simulink model "torqueWalkingR2017a"  (Simulink 9.0)
settings: Solver=FixedStepDiscrete  StartTime=0.0  StopTime=Config.t_end  FixedStep=Config.t_step  RelTol=1e-3  EnableMultiTasking=on
InitFcn:
  | cd(fileparts(which(bdroot)));
  | initTorqueWalking;
StopFcn:
  | cd(fileparts(which(bdroot)));
  | disp_early_termination
undefined symbols (not defined in the file or in its folder): biasVectorConstraint_feet, Config, CONFIG, ConstraintMatrix_feet, DiscIntNeverNeededParam, Gains, ROBOT_DOF, Sat
libraries: WBToolboxLibrary x113, commchan3 x2, simulink x2
(part 4 of 4)

== system torqueWalkingR2017a/Robot State and References/Smooth References /Smooth Reference Orientations/Compute Smoothed Ref Orientations ==
  w_R_LFoot_des : Inport
  w_R_RFoot_des : Inport  Port=2
  w_R_rot_task_des : Inport  Port=3
  w_R_LHand_des : Inport  Port=4
  w_R_RHand_des : Inport  Port=5
  omega_LFoot : Inport  Port=6
  omega_RFoot : Inport  Port=7
  omega_rot_task : Inport  Port=8
  omega_LHand : Inport  Port=9
  omega_RHand : Inport  Port=10
  Compute Rotation Matrix Derivative : MATLAB Function  TreatAsAtomicUnit=on
  Discrete-Time Integrator{1..5} (5 alike) : DiscreteIntegrator  InitialConditionSource=external  InitialCondition=zeros(3,1)  InitialConditionSetting=State (most efficient)  SampleTime=Config.t_step  ICPrevOutput=DiscIntNeverNeededParam  ICPrevScaledInput=DiscIntNeverNeededParam
  holder {,1..4} (5 alike) : WBToolboxLibrary/Utilities/holder 
      settings: SourceProductName=Whole Body Toolbox
  w_R_LFoot : Outport
  w_R_RFoot : Outport  Port=2
  w_R_rot_task : Outport  Port=3
  w_R_LHand : Outport  Port=4
  w_R_RHand : Outport  Port=5
  wires:
  "holder "/1 -> Discrete-Time Integrator2/2
  holder 2/1 -> Discrete-Time Integrator5/2
  holder 1/1 -> Discrete-Time Integrator1/2
  Compute Rotation Matrix Derivative/1(RDot_LFoot) -> Discrete-Time Integrator2/1
  Compute Rotation Matrix Derivative/2(RDot_RFoot) -> Discrete-Time Integrator5/1
  Compute Rotation Matrix Derivative/3(RDot_rot_task) -> Discrete-Time Integrator1/1
  w_R_LFoot_des/1 -> "holder "/1
  w_R_RFoot_des/1 -> holder 2/1
  w_R_rot_task_des/1 -> holder 1/1
  Discrete-Time Integrator2/1 -> w_R_LFoot/1, Compute Rotation Matrix Derivative/6(w_R_LFoot)
  Discrete-Time Integrator1/1 -> w_R_rot_task/1, Compute Rotation Matrix Derivative/8(w_R_rot_task)
  omega_LFoot/1 -> Compute Rotation Matrix Derivative/1(omega_LFoot)
  omega_RFoot/1 -> Compute Rotation Matrix Derivative/2(omega_RFoot)
  omega_rot_task/1 -> Compute Rotation Matrix Derivative/3(omega_rot_task)
  Discrete-Time Integrator5/1 -> w_R_RFoot/1, Compute Rotation Matrix Derivative/7(w_R_RFoot)
  omega_LHand/1 -> Compute Rotation Matrix Derivative/4(omega_LHand)
  omega_RHand/1 -> Compute Rotation Matrix Derivative/5(omega_RHand)
  Discrete-Time Integrator4/1 -> w_R_RHand/1, Compute Rotation Matrix Derivative/10(w_R_RHand)
  Discrete-Time Integrator3/1 -> w_R_LHand/1, Compute Rotation Matrix Derivative/9(w_R_LHand)
  w_R_RHand_des/1 -> holder 4/1
  w_R_LHand_des/1 -> holder 3/1
  Compute Rotation Matrix Derivative/5(RDot_RHand) -> Discrete-Time Integrator4/1
  Compute Rotation Matrix Derivative/4(RDot_LHand) -> Discrete-Time Integrator3/1
  holder 4/1 -> Discrete-Time Integrator4/2
  holder 3/1 -> Discrete-Time Integrator3/2

== system torqueWalkingR2017a/Robot State and References/State Machines/Compute Feet to Base Link Transforms/LFoot to base link transform  ==
  s : Inport
  inertial : Inport  Port=2
  w_H_link : Inport  Port=3
  w_H_base_fixed : Inport  Port=4
  Fixed base to imu transform : WBToolboxLibrary/wholeBodyModel/Kinematics/Forward Kinematics  frameName=Frames.IMU
      settings: SourceProductName=Whole Body Toolbox
  Fixed base to root link transform : WBToolboxLibrary/wholeBodyModel/Kinematics/Forward Kinematics  frameName=Frames.BASE_LINK
      settings: SourceProductName=Whole Body Toolbox
  Inv\* : Product  Inputs=/*  Multiplication=Matrix(*)
  "Inv\\*  " : Product  Inputs=/*  Multiplication=Matrix(*)
  Neck Position : WBToolboxLibrary/Utilities/Yarp Read  portName=Ports.NECK_POS  signalSize=6  timeout=0.5  blocking=off  timestamp=off  autoconnect=on  errorOnConnection=off
      settings: SourceProductName=Whole Body Toolbox
  Switch6 : Switch  Criteria=u2 > Threshold
  USE_IMU4EST_BASE : Constant  Value=Config.USE_IMU4EST_BASE
  fromImuToHomogeousTransformFCN : MATLAB Function  TreatAsAtomicUnit=on
  holder 1 : WBToolboxLibrary/Utilities/holder 
      settings: SourceProductName=Whole Body Toolbox
  holder 2 : WBToolboxLibrary/Utilities/holder 
      settings: SourceProductName=Whole Body Toolbox
  neck transform : Subsystem
  link_H_b : Outport
  wires:
  Switch6/1 -> link_H_b/1
  "Inv\\*  "/1 -> Switch6/3, fromImuToHomogeousTransformFCN/3(link_H_base)  "link_H_root"
  USE_IMU4EST_BASE/1 -> Switch6/2
  Inv\*/1 -> fromImuToHomogeousTransformFCN/1(imu_H_link), holder 1/1  "imu_H_link"
  holder 2/1 -> fromImuToHomogeousTransformFCN/4(inertial_0)
  Fixed base to imu transform/1 -> Inv\*/1
  holder 1/1 -> fromImuToHomogeousTransformFCN/2(imu_H_link_0)
  s/1 -> Fixed base to imu transform/2, Fixed base to root link transform/2
  fromImuToHomogeousTransformFCN/1(w_H_b) -> Switch6/1
  Fixed base to root link transform/1 -> "Inv\\*  "/2
  inertial/1 -> holder 2/1, fromImuToHomogeousTransformFCN/5(inertial)
  Neck Position/1 -> neck transform/1(neck port)
  neck transform/1(neck position) -> fromImuToHomogeousTransformFCN/6(neck_pos)
  w_H_link/1 -> "Inv\\*  "/1, Inv\*/2
  w_H_base_fixed/1 -> Fixed base to root link transform/1, Fixed base to imu transform/1

== system torqueWalkingR2017a/Robot State and References/State Machines/Compute Feet to Base Link Transforms/RFoot to base link transform ==
  s : Inport
  inertial : Inport  Port=2
  w_H_link : Inport  Port=3
  w_H_base_fixed : Inport  Port=4
  Fixed base to imu transform : WBToolboxLibrary/wholeBodyModel/Kinematics/Forward Kinematics  frameName=Frames.IMU
      settings: SourceProductName=Whole Body Toolbox
  Fixed base to root link transform : WBToolboxLibrary/wholeBodyModel/Kinematics/Forward Kinematics  frameName=Frames.BASE_LINK
      settings: SourceProductName=Whole Body Toolbox
  Inv\* : Product  Inputs=/*  Multiplication=Matrix(*)
  "Inv\\*  " : Product  Inputs=/*  Multiplication=Matrix(*)
  Neck Position : WBToolboxLibrary/Utilities/Yarp Read  portName=Ports.NECK_POS  signalSize=6  timeout=0.5  blocking=off  timestamp=off  autoconnect=on  errorOnConnection=off
      settings: SourceProductName=Whole Body Toolbox
  Switch6 : Switch  Criteria=u2 > Threshold
  USE_IMU4EST_BASE : Constant  Value=Config.USE_IMU4EST_BASE
  fromImuToHomogeousTransformFCN : MATLAB Function  TreatAsAtomicUnit=on
  holder 1 : WBToolboxLibrary/Utilities/holder 
      settings: SourceProductName=Whole Body Toolbox
  holder 2 : WBToolboxLibrary/Utilities/holder 
      settings: SourceProductName=Whole Body Toolbox
  neck transform : Subsystem
  link_H_b : Outport
  wires:
  Switch6/1 -> link_H_b/1
  "Inv\\*  "/1 -> Switch6/3, fromImuToHomogeousTransformFCN/3(link_H_base)  "link_H_root"
  USE_IMU4EST_BASE/1 -> Switch6/2
  Inv\*/1 -> fromImuToHomogeousTransformFCN/1(imu_H_link), holder 1/1  "imu_H_link"
  holder 2/1 -> fromImuToHomogeousTransformFCN/4(inertial_0)
  Fixed base to imu transform/1 -> Inv\*/1
  holder 1/1 -> fromImuToHomogeousTransformFCN/2(imu_H_link_0)
  s/1 -> Fixed base to imu transform/2, Fixed base to root link transform/2
  fromImuToHomogeousTransformFCN/1(w_H_b) -> Switch6/1
  Fixed base to root link transform/1 -> "Inv\\*  "/2
  inertial/1 -> holder 2/1, fromImuToHomogeousTransformFCN/5(inertial)
  Neck Position/1 -> neck transform/1(neck port)
  neck transform/1(neck position) -> fromImuToHomogeousTransformFCN/6(neck_pos)
  w_H_link/1 -> "Inv\\*  "/1, Inv\*/2
  w_H_base_fixed/1 -> Fixed base to root link transform/1, Fixed base to imu transform/1

== system torqueWalkingR2017a/Robot State and References/State Machines/Compute State Velocity/Feet Jacobians ==
  s : Inport
  w_H_b : Inport  Port=2
  Jacobian LFoot : WBToolboxLibrary/wholeBodyModel/Jacobians/Jacobian  frameName=Frames.LEFT_FOOT
      settings: SourceProductName=Whole Body Toolbox
  Jacobian RFoot : WBToolboxLibrary/wholeBodyModel/Jacobians/Jacobian  frameName=Frames.RIGHT_FOOT
      settings: SourceProductName=Whole Body Toolbox
  J_LFoot : Outport
  J_RFoot : Outport  Port=2
  wires:
  Jacobian LFoot/1 -> J_LFoot/1
  Jacobian RFoot/1 -> J_RFoot/1
  w_H_b/1 -> Jacobian RFoot/1, Jacobian LFoot/1
  s/1 -> Jacobian LFoot/2, Jacobian RFoot/2

== system torqueWalkingR2017a/Robot State and References/State Machines/Select the Current State and References/task position and orientation ==
  s : Inport
  w_H_b : Inport  Port=2
  CoM : WBToolboxLibrary/wholeBodyModel/Kinematics/Forward Kinematics  frameName=Frames.COM
      settings: SourceProductName=Whole Body Toolbox
  LArm : WBToolboxLibrary/wholeBodyModel/Kinematics/Forward Kinematics  frameName=Frames.LEFT_HAND
      settings: SourceProductName=Whole Body Toolbox
  LFoot : WBToolboxLibrary/wholeBodyModel/Kinematics/Forward Kinematics  frameName=Frames.LEFT_FOOT
      settings: SourceProductName=Whole Body Toolbox
  RArm : WBToolboxLibrary/wholeBodyModel/Kinematics/Forward Kinematics  frameName=Frames.RIGHT_HAND
      settings: SourceProductName=Whole Body Toolbox
  RFoot : WBToolboxLibrary/wholeBodyModel/Kinematics/Forward Kinematics  frameName=Frames.RIGHT_FOOT
      settings: SourceProductName=Whole Body Toolbox
  rotational task : WBToolboxLibrary/wholeBodyModel/Kinematics/Forward Kinematics  frameName=Frames.ROT_TASK_LINK
      settings: SourceProductName=Whole Body Toolbox
  w_H_l_sole : Outport
  w_H_r_sole : Outport  Port=2
  w_H_CoM : Outport  Port=3
  w_H_rot_task : Outport  Port=4
  w_H_l_hand : Outport  Port=5
  w_H_r_hand : Outport  Port=6
  wires:
  s/1 -> RArm/2, LArm/2, rotational task/2, CoM/2, RFoot/2, LFoot/2
  w_H_b/1 -> RArm/1, LArm/1, rotational task/1, CoM/1, LFoot/1, RFoot/1
  CoM/1 -> w_H_CoM/1
  LFoot/1 -> w_H_l_sole/1
  RFoot/1 -> w_H_r_sole/1
  rotational task/1 -> w_H_rot_task/1
  LArm/1 -> w_H_l_hand/1
  RArm/1 -> w_H_r_hand/1

== system torqueWalkingR2017a/Robot State and References/State Machines/Compute Feet to Base Link Transforms/LFoot to base link transform /neck transform ==
  neck port : Inport
  Constant : Constant  Value=zeros(3,1)
  Gain : Gain  Gain=pi/180
  Selector1 : Selector  InputPortWidth=6  IndexOptions=Index vector (dialog)  Indices=[1:3]  OutputSizes=1
  Switch : Switch  Criteria=u2 > Threshold
  USE_IMU4EST_BASE1 : Constant  Value=Config.CORRECT_IMU_WITH_NECK_POS
  neck position : Outport
  wires:
  neck port/1 -> Gain/1
  USE_IMU4EST_BASE1/1 -> Switch/2
  Switch/1 -> neck position/1
  Gain/1 -> Selector1/1
  Constant/1 -> Switch/3
  Selector1/1 -> Switch/1  "neck pos"

== system torqueWalkingR2017a/Robot State and References/State Machines/Compute Feet to Base Link Transforms/RFoot to base link transform/neck transform ==
  neck port : Inport
  Constant : Constant  Value=zeros(3,1)
  Gain : Gain  Gain=pi/180
  Selector1 : Selector  InputPortWidth=6  IndexOptions=Index vector (dialog)  Indices=[1:3]  OutputSizes=1
  Switch : Switch  Criteria=u2 > Threshold
  USE_IMU4EST_BASE1 : Constant  Value=Config.CORRECT_IMU_WITH_NECK_POS
  neck position : Outport
  wires:
  neck port/1 -> Gain/1
  USE_IMU4EST_BASE1/1 -> Switch/2
  Switch/1 -> neck position/1
  Gain/1 -> Selector1/1
  Constant/1 -> Switch/3
  Selector1/1 -> Switch/1  "neck pos"

== matlab function Dynamics and Kinematics/Initial Conditions/compute state velocity/Compute Base Velocity ==
  data: J_LeftFoot input double; J_RightFoot input double; feetInContact input double; nu_b output double; sDot input double; Sat parameter double
function nu_b = computeBaseVelocityFCN(J_LeftFoot, J_RightFoot, feetInContact, sDot, Sat)

    nu_b = computeBaseVelocity(J_LeftFoot, J_RightFoot, feetInContact, sDot, Sat);
end

== matlab function Balancing Controller (Reactive QP control)/Balancing Controller Function ==
  data: feetInContact input double; M input double; Hessian output double; h input double; J input double; impedances input double; dampings input double; s input double; sDot input double; s_sDot_sDDot_des input double; acc_task_star input double; JDot_nu input double; ConstraintsMatrix_feet input double; biasVectorConstraint_feet input double; w_H_l_sole input double; w_H_r_sole input double; gradient output double; ConstraintMatrix_equality output double; biasVectorConstraint_equality output double; ConstraintMatrix_inequality output double; biasVectorConstraint_inequality output double; Sat parameter double; Config parameter double; ROBOT_DOF parameter double
function [Hessian,gradient,ConstraintMatrix_equality,biasVectorConstraint_equality, ...
          ConstraintMatrix_inequality,biasVectorConstraint_inequality] = ...
          balancingControllerFCN(feetInContact, M, h, J, impedances, ...
                                 dampings, s, sDot, s_sDot_sDDot_des, acc_task_star, ...
                                 JDot_nu, ConstraintsMatrix_feet, biasVectorConstraint_feet, ...
                                 w_H_l_sole, w_H_r_sole, Sat, Config, ROBOT_DOF)
                          

    [Hessian,gradient,ConstraintMatrix_equality,biasVectorConstraint_equality, ...
     ConstraintMatrix_inequality,biasVectorConstraint_inequality] = ...
         balancingController(feetInContact, M, h, J, impedances, ...
                                dampings, s, sDot, s_sDot_sDDot_des, acc_task_star, ...
                                JDot_nu, ConstraintsMatrix_feet, biasVectorConstraint_feet, ...
                                w_H_l_sole, w_H_r_sole, Sat, Config, ROBOT_DOF);                         
end

== matlab function Dynamics and Kinematics/Inverse Kinematics/Compute tasks accelerations ==
  data: pose_vel_acc_LFoot_des input double; pose_vel_acc_RFoot_des input double; pos_vel_acc_CoM_des input double; acc_task_star output double; orient_vel_acc_rot_task_des input double; pose_vel_acc_LHand_des input double; pose_vel_acc_RHand_des input double; pose_vel_LFoot input double; pose_vel_RFoot input double; pos_vel_CoM input double; orient_vel_rot_task input double; pose_vel_LHand input double; pose_vel_RHand input double; Kp_Kd_LFoot input double; Kp_Kd_RFoot input double; Kp_Kd_CoM input double; Kp_Kd_rot_task input double; Kp_Kd_LHand input double; Kp_Kd_RHand input double; feetInContact input double; Sat parameter double
function acc_task_star = setTasksAccelerationsFCN(pose_vel_acc_LFoot_des, pose_vel_acc_RFoot_des, pos_vel_acc_CoM_des, orient_vel_acc_rot_task_des, pose_vel_acc_LHand_des,pose_vel_acc_RHand_des, ...
                                                  pose_vel_LFoot, pose_vel_RFoot, pos_vel_CoM, orient_vel_rot_task, pose_vel_LHand, pose_vel_RHand, ...
                                                  Kp_Kd_LFoot, Kp_Kd_RFoot, Kp_Kd_CoM, Kp_Kd_rot_task, Kp_Kd_LHand, Kp_Kd_RHand,...
                                                  feetInContact, Sat) 

    acc_task_star = setTasksAccelerations(pos_vel_acc_CoM_des, pose_vel_acc_LFoot_des, pose_vel_acc_RFoot_des, orient_vel_acc_rot_task_des, pose_vel_acc_LHand_des,pose_vel_acc_RHand_des, ...
                                          pos_vel_CoM, pose_vel_LFoot, pose_vel_RFoot, orient_vel_rot_task, pose_vel_LHand, pose_vel_RHand, ...
                                          Kp_Kd_CoM, Kp_Kd_LFoot, Kp_Kd_RFoot, Kp_Kd_rot_task, Kp_Kd_LHand, Kp_Kd_RHand,...
                                          feetInContact, Sat) ; 
                                      
                                      
end

== matlab function Dynamics and Kinematics/Inverse Kinematics/ComputeTasksPoseAndVelocity/Compose Task Pose and Velocity ==
  data: vel_LFoot input double; vel_RFoot input double; pose_vel_LFoot output double; pose_vel_RFoot output double; vel_CoM input double; vel_rot_task input double; vel_LHand input double; vel_RHand input double; w_H_l_sole input double; w_H_r_sole input double; pos_vel_CoM output double; orient_vel_rot_task output double; w_H_CoM input double; w_H_rot_task input double; w_H_l_hand input double; w_H_r_hand input double; pose_vel_LHand output double; pose_vel_RHand output double
function [pose_vel_LFoot, pose_vel_RFoot, pos_vel_CoM, orient_vel_rot_task, pose_vel_LHand, pose_vel_RHand] = ...
             composeTaskPoseAndVelocityFCN(vel_LFoot, vel_RFoot, vel_CoM, vel_rot_task, vel_LHand, vel_RHand, ...
                                           w_H_l_sole, w_H_r_sole, w_H_CoM, w_H_rot_task, w_H_l_hand, w_H_r_hand)
                                                                                                                              
    [pos_vel_CoM, pose_vel_LFoot, pose_vel_RFoot, orient_vel_rot_task, pose_vel_LHand, pose_vel_RHand] = ...
        composeTaskPoseAndVelocity(vel_CoM, vel_LFoot, vel_RFoot, vel_rot_task, vel_LHand, vel_RHand, ...
                                   w_H_CoM, w_H_l_sole, w_H_r_sole, w_H_rot_task, w_H_l_hand, w_H_r_hand);
end

== matlab function Dynamics and Kinematics/Inverse Kinematics/QP-Based Inverse Kinematics/Compute QP Hessian, gradient and constraints  ==
  data: s input double; nu input double; s_sDot_sDDot_ref input double; Hessian output double; impedances input double; dampings input double; J input double; JDot_nu input double; acc_task_star input double; feetInContact input double; gradient output double; ConstraintMatrix output double; biasVectorConstraint output double; Config parameter double; Sat parameter double
function [Hessian, gradient, ConstraintMatrix, biasVectorConstraint] = ...
             computeQPHessianAndConstraintsFCN(s, nu, s_sDot_sDDot_ref, impedances, dampings, J, JDot_nu, acc_task_star, feetInContact, Config, Sat)
         
    [Hessian, gradient, ConstraintMatrix, biasVectorConstraint] = ...
        computeQPHessianAndConstraints(s, nu, s_sDot_sDDot_ref, impedances, dampings, J, JDot_nu, acc_task_star, feetInContact, Sat, Config);
end

== matlab function Dynamics and Kinematics/Task Accelerations/Compute tasks accelerations ==
  data: pos_vel_acc_CoM_des input double; acc_task_star output double; pose_vel_acc_LFoot_des input double; pose_vel_acc_RFoot_des input double; orient_vel_acc_rot_task_des input double; pose_vel_acc_LHand_des input double; pose_vel_acc_RHand_des input double; pos_vel_CoM input double; pose_vel_LFoot input double; pose_vel_RFoot input double; orient_vel_rot_task input double; pose_vel_LHand input double; pose_vel_RHand input double; Kp_Kd_CoM input double; Kp_Kd_LFoot input double; Kp_Kd_RFoot input double; Kp_Kd_rot_task input double; Kp_Kd_LHand input double; Kp_Kd_RHand input double; feetInContact input double; Sat parameter double
function acc_task_star = setTasksAccelerationsFCN(pos_vel_acc_CoM_des, pose_vel_acc_LFoot_des, pose_vel_acc_RFoot_des, orient_vel_acc_rot_task_des, pose_vel_acc_LHand_des,pose_vel_acc_RHand_des, ...
                                                  pos_vel_CoM, pose_vel_LFoot, pose_vel_RFoot, orient_vel_rot_task, pose_vel_LHand, pose_vel_RHand, ...
                                                  Kp_Kd_CoM, Kp_Kd_LFoot, Kp_Kd_RFoot, Kp_Kd_rot_task, Kp_Kd_LHand, Kp_Kd_RHand,...
                                                  feetInContact, Sat) 

    acc_task_star = setTasksAccelerations(pos_vel_acc_CoM_des, pose_vel_acc_LFoot_des, pose_vel_acc_RFoot_des, orient_vel_acc_rot_task_des, pose_vel_acc_LHand_des,pose_vel_acc_RHand_des, ...
                                          pos_vel_CoM, pose_vel_LFoot, pose_vel_RFoot, orient_vel_rot_task, pose_vel_LHand, pose_vel_RHand, ...
                                          Kp_Kd_CoM, Kp_Kd_LFoot, Kp_Kd_RFoot, Kp_Kd_rot_task, Kp_Kd_LHand, Kp_Kd_RHand,...
                                          feetInContact, Sat);

end

== matlab function Dynamics and Kinematics/Task Accelerations/ComputeTasksPoseAndVelocity/Compose Task Pose and Velocity ==
  data: vel_CoM input double; vel_LFoot input double; vel_RFoot input double; vel_rot_task input double; vel_LHand input double; vel_RHand input double; pos_vel_CoM output double; pose_vel_LFoot output double; pose_vel_RFoot output double; orient_vel_rot_task output double; w_H_CoM input double; w_H_l_sole input double; w_H_r_sole input double; w_H_rot_task input double; w_H_l_hand input double; w_H_r_hand input double; pose_vel_LHand output double; pose_vel_RHand output double
function [pos_vel_CoM, pose_vel_LFoot, pose_vel_RFoot, orient_vel_rot_task, pose_vel_LHand, pose_vel_RHand] = ...
             composeTaskPoseAndVelocityFCN(vel_CoM, vel_LFoot, vel_RFoot, vel_rot_task, vel_LHand, vel_RHand, ...
                                           w_H_CoM, w_H_l_sole, w_H_r_sole, w_H_rot_task, w_H_l_hand, w_H_r_hand)
                                                                                                                              
    [pos_vel_CoM, pose_vel_LFoot, pose_vel_RFoot, orient_vel_rot_task, pose_vel_LHand, pose_vel_RHand] = ...
        composeTaskPoseAndVelocity(vel_CoM, vel_LFoot, vel_RFoot, vel_rot_task, vel_LHand, vel_RHand, ...
                                   w_H_CoM, w_H_l_sole, w_H_r_sole, w_H_rot_task, w_H_l_hand, w_H_r_hand);
end

== matlab function Robot State and References/Gain Scheduling/Gain Scheduling Function ==
  data: state input double; Kp_CoM output double; Kd_CoM output double; Kp_LFoot output double; Kd_LFoot output double; Kp_RFoot output double; Kd_RFoot output double; Kp_rot_task output double; Kd_rot_task output double; Kp_LHand output double; Kd_LHand output double; Kp_RHand output double; Kd_RHand output double; impedances output double; dampings output double; Gains parameter double; smoothingTimeGains output double; Config parameter double
function [Kp_CoM, Kd_CoM, Kp_LFoot, Kd_LFoot, Kp_RFoot, Kd_RFoot, Kp_rot_task, Kd_rot_task, Kp_LHand, Kd_LHand, Kp_RHand, Kd_RHand, impedances, dampings, smoothingTimeGains] = ...
             gainSchedulingFCN(state,Gains,Config)

    [Kp_CoM, Kd_CoM, Kp_LFoot, Kd_LFoot, Kp_RFoot, Kd_RFoot, Kp_rot_task, Kd_rot_task, Kp_LHand, Kd_LHand, Kp_RHand, Kd_RHand, impedances, dampings, smoothingTimeGains] = ...
        gainScheduling(state,Gains,Config);
end

== matlab function Robot State and References/Smooth References /Smooth Reference Orientations/Compute Ref Ang Velocities and Accelerations/Compute Reference Angular Accelerations ==
  data: w_R_LFoot_des input double; w_R_RFoot_des input double; w_R_rot_task_des input double; w_R_LHand_des input double; w_R_RHand_des input double; w_R_LFoot input double; w_R_RFoot input double; omegaDot_LFoot output double; omegaDot_RFoot output double; omegaDot_rot_task output double; w_R_rot_task input double; w_R_LHand input double; w_R_RHand input double; state input double; omega_LFoot input double; omega_RFoot input double; omega_rot_task input double; omega_LHand input double; omega_RHand input double; Config parameter double; omegaDot_LHand output double; omegaDot_RHand output double
function [omegaDot_LFoot, omegaDot_RFoot, omegaDot_rot_task, omegaDot_LHand, omegaDot_RHand] = computeRefAngAccelerationFCN(w_R_LFoot_des, w_R_RFoot_des, w_R_rot_task_des, w_R_LHand_des, w_R_RHand_des, ...
                                                                                            w_R_LFoot, w_R_RFoot, w_R_rot_task, w_R_LHand, w_R_RHand, ...
                                                                                            state, omega_LFoot, omega_RFoot, omega_rot_task, omega_LHand, omega_RHand, Config)
         
    % Compute reference angular accelerations given a desired rotation matrix
    omegaDot_LFoot     = rotationalPID(w_R_LFoot, omega_LFoot, w_R_LFoot_des, zeros(3,1), zeros(3,1), ...
                                       Config.LFoot_Kp_smoothing(state), Config.LFoot_Kd_smoothing(state));
                                   
    omegaDot_RFoot     = rotationalPID(w_R_RFoot, omega_RFoot, w_R_RFoot_des, zeros(3,1), zeros(3,1), ...
                                       Config.RFoot_Kp_smoothing(state), Config.RFoot_Kd_smoothing(state));
                                   
    omegaDot_rot_task  = rotationalPID(w_R_rot_task, omega_rot_task, w_R_rot_task_des, zeros(3,1), zeros(3,1), ...
                                       Config.rot_task_Kp_smoothing(state), Config.rot_task_Kd_smoothing(state));

    omegaDot_LHand     = rotationalPID(w_R_LHand, omega_LHand, w_R_LHand_des, zeros(3,1), zeros(3,1), ...
                                       Config.LHand_Kp_smoothing(state), Config.LHand_Kd_smoothing(state));
                                   
    omegaDot_RHand     = rotationalPID(w_R_RHand, omega_RHand, w_R_RHand_des, zeros(3,1), zeros(3,1), ...
                                       Config.RHand_Kp_smoothing(state), Config.RHand_Kd_smoothing(state));

end

== matlab function Robot State and References/State Machines/Select the Current State and References/STATE MACHINES ==
  data: w_H_b output double; feetInContact output double; s_0 input double; w_H_LFoot input double; w_H_LFoot_0 input double; w_H_RFoot input double; w_H_RFoot_0 input double; w_H_CoM input double; w_H_CoM_0 input double; w_H_rot_task_0 input double; w_H_LHand_0 input double; w_H_RHand_0 input double; LFoot_H_b input double; RFoot_H_b input double; LFoot_wrench input double; RFoot_wrench input double; t input double; state output double; references_LFoot output double; references_RFoot output double; references_CoM output double; references_rot_task output double; references_LHand output double; references_RHand output double; references_s output double; Config parameter double; Sat parameter double
function [w_H_b, feetInContact, state, references_LFoot, references_RFoot, references_CoM, ...
          references_rot_task, references_LHand, references_RHand, references_s] = stateMachinesFCN ...
             (s_0, w_H_LFoot, w_H_LFoot_0, w_H_RFoot, w_H_RFoot_0, w_H_CoM, w_H_CoM_0, w_H_rot_task_0, ...
              w_H_LHand_0, w_H_RHand_0, LFoot_H_b, RFoot_H_b, LFoot_wrench, RFoot_wrench, t, Config, Sat)

    [w_H_b, feetInContact, state, references_LFoot, references_RFoot, references_CoM, ...
     references_rot_task, references_LHand, references_RHand, references_s] = stateMachineWalkingInPlace ...
        (s_0, w_H_LFoot, w_H_LFoot_0, w_H_RFoot, w_H_RFoot_0, w_H_CoM, w_H_CoM_0, w_H_rot_task_0, ...
         w_H_LHand_0, w_H_RHand_0, LFoot_H_b, RFoot_H_b, LFoot_wrench, RFoot_wrench, t, Config, Sat);

end

== matlab function Robot State and References/State Machines/Compute Feet to Base Link Transforms/LFoot to base link transform /fromImuToHomogeousTransformFCN ==
  data: imu_H_link input double; imu_H_link_0 input double; link_H_base input double; inertial_0 input double; inertial input double; neck_pos input double; w_H_b output double; Config parameter double
function w_H_b = worldToBaseTransformWithIMUFCN(imu_H_link,imu_H_link_0,link_H_base,inertial_0,inertial,neck_pos,Config)

    w_H_b = worldToBaseTransformWithIMU(imu_H_link,imu_H_link_0,link_H_base,inertial_0,inertial,neck_pos,Config);

end

== matlab function Robot State and References/Smooth References /Smooth Reference Orientations/Compute Smoothed Ref Orientations/Compute Rotation Matrix Derivative ==
  data: RDot_LFoot output double; RDot_RFoot output double; RDot_rot_task output double; omega_LFoot input double; omega_RFoot input double; omega_rot_task input double; omega_LHand input double; omega_RHand input double; w_R_LFoot input double; w_R_RFoot input double; w_R_rot_task input double; w_R_LHand input double; w_R_RHand input double; RDot_LHand output double; RDot_RHand output double
function [RDot_LFoot, RDot_RFoot, RDot_rot_task, RDot_LHand, RDot_RHand] = rotationDerivativeFromAngVelFCN(omega_LFoot, omega_RFoot, omega_rot_task, omega_LHand, omega_RHand, ... 
                                                                                   w_R_LFoot, w_R_RFoot, w_R_rot_task, w_R_LHand, w_R_RHand)
         
    % Compute the rotation matrix derivative given the angular velocity
    RDot_LFoot     = rotationDerivativeFromAngVel(omega_LFoot,w_R_LFoot);
    RDot_RFoot     = rotationDerivativeFromAngVel(omega_RFoot,w_R_RFoot);
    RDot_rot_task  = rotationDerivativeFromAngVel(omega_rot_task, w_R_rot_task); 
    RDot_LHand     = rotationDerivativeFromAngVel(omega_LHand,w_R_LHand);
    RDot_RHand     = rotationDerivativeFromAngVel(omega_RHand,w_R_RHand);
end

== matlab function Robot State and References/State Machines/Compute Feet to Base Link Transforms/RFoot to base link transform/fromImuToHomogeousTransformFCN ==
  data: imu_H_link input double; imu_H_link_0 input double; link_H_base input double; inertial_0 input double; inertial input double; neck_pos input double; w_H_b output double; Config parameter double
function w_H_b = worldToBaseTransformWithIMUFCN(imu_H_link,imu_H_link_0,link_H_base,inertial_0,inertial,neck_pos,Config)

    w_H_b = worldToBaseTransformWithIMU(imu_H_link,imu_H_link_0,link_H_base,inertial_0,inertial,neck_pos,Config);

end

== matlab function Robot State and References/State Machines/Compute State Velocity/Compute Base Velocity ==
  data: J_LeftFoot input double; J_RightFoot input double; feetInContact input double; nu_b output double; sDot input double; Sat parameter double
function nu_b = computeBaseVelocityFCN(J_LeftFoot, J_RightFoot, feetInContact, sDot, Sat)

    nu_b = computeBaseVelocity(J_LeftFoot, J_RightFoot, feetInContact, sDot, Sat);
end

== matlab function Dynamics and Kinematics/Inverse Kinematics/QP-Based Inverse Kinematics/inverse kinematics integration/Rewrite Base Pose as transformation matrix ==
  data: pose_b input double; w_H_b output double
function  w_H_b = fromPosQuatToTransfMatrFCN(pose_b) 

    % converts the base pose from a position + quaternion representation 
    % to a tranformation matrix
    w_H_b = fromPosQuatToTransfMatr(pose_b);
end

== matlab function Dynamics and Kinematics/Inverse Kinematics/QP-Based Inverse Kinematics/inverse kinematics integration/Compute Base Pose Derivative ==
  data: pose_b input double; nu_b input double; pose_bDot output double
function pose_bDot = basePoseDerivativeFCN(pose_b,nu_b)

    % time derivative of the floating base pose
    pose_bDot = basePoseDerivative(nu_b, pose_b);
end

== matlab function Robot State and References/Smooth References /Smooth Reference Positions/Configure Settling Times ==
  data: state input double; Config parameter double; smoothingTime_CoM output double; smoothingTime_LFoot output double; smoothingTime_RFoot output double; smoothingTime_joints output double; smoothingTime_LHand output double; smoothingTime_RHand output double
function [smoothingTime_CoM, smoothingTime_LFoot, smoothingTime_RFoot, smoothingTime_joints, smoothingTime_LHand, smoothingTime_RHand] = setSmoothingTimesFCN(state,Config)

    [smoothingTime_CoM, smoothingTime_LFoot, smoothingTime_RFoot, smoothingTime_joints, smoothingTime_LHand, smoothingTime_RHand] = setSmoothingTimes(state,Config);

end

== matlab function Dynamics and Kinematics/Inverse Kinematics/QP-Based Inverse Kinematics/inverse kinematics integration/Rewrite Base Pose as pos+quat ==
  data: w_H_b_0 input double; pose_b_0 output double
function pose_b_0 = fromTransfMatrixToPosQuatFCN(w_H_b_0)

    % converts the floating base pose expressed in terms of transformation
    % matrix into position + quaternion representation 
    pose_b_0 = fromTransfMatrixToPosQuat(w_H_b_0);

end

== matlab function Disturbances for learnoptim_wbc/Apply external wrench/Apply external wrench on iCub chest ==
  data: external_force parameter double; time input double
function sendExternalWrench(external_force, time)

coder.extrinsic('system') 
coder.extrinsic('num2str')
%how to send a command to apply external force:
%system('echo "chest 20 0 0 0 0 0 1" | yarp rpc /icubSim/applyExternalWrench/rpc:i');

%check if the current time corresponds to a time at which a wrench should
%be applied
index = find(external_force.time_of_application == time);

%If a force should be applied at the current time,
%it can be found at the index "index"
if index
    link     = external_force.link;    
    wrench   = [num2str(external_force.wrench(index,1)) ' ' num2str(external_force.wrench(index,2)) ' ' ...
                num2str(external_force.wrench(index,3)) ' ' num2str(external_force.wrench(index,4)) ' ' ...
                num2str(external_force.wrench(index,5)) ' ' num2str(external_force.wrench(index,6))];
    duration = num2str(external_force.duration(index));
    
    disp('applying external wrench');
    force_to_apply = ['"' link ' ' wrench ' ' duration '"'];
    system(['echo ' force_to_apply ' | yarp rpc /icubSim/applyExternalWrench/rpc:i']);
end

== matlab function Dynamics and Kinematics/Compute Dynamic and Kinematic Quantities/Mass Matrix and Bias Forces/Add motors reflected inertias/Add motor reflected inertias ==
  data: M input double; M_with_inertia output double; Config parameter double
function M_with_inertia = addMotorsInertiaFCN(M,Config)

    M_with_inertia = addMotorsInertia(M,Config);

end

== matlab function Subsystem/compute ZMP ==
  data: f_lFoot input double; f_rFoot input double; ZMP output double; pose_lFoot input double; orient_lFoot input double; pose_rFoot input double; orient_rFoot input double; Sat parameter double; Config parameter double; supportPolygon output double; zmpErr output double
function [ZMP, supportPolygon,zmpErr] = ZMP(f_lFoot, f_rFoot, pose_lFoot, orient_lFoot, pose_rFoot, orient_rFoot, Sat, Config)

% % Compute the coordinates of the ZMP
% % Compute the coordinates of the support polygon
% %
% %           right_foot      left_foot
% %         C  _______  B   C' _______ B'          
% %           |       |       |       |   Y_w
% %           |       |       |   ---------->
% %           |       |       |   |   |
% %         D |_______| A   D'|___|__ | A'
% %                               |
% %                           X_w |
% %                               v
% % 
% % input Config.footSize = [xMin, xMax]
% %                         [yMin, yMax] 
% %                            
% % output supportPolygon = [xMin, xMax]
% %                         [yMin, yMax]

%Re-organize foot size into min/max coordinates
foot_xMin    = Config.footSize(1,1);
foot_xMax    = Config.footSize(1,2);
foot_yMin    = Config.footSize(2,1);
foot_yMax    = Config.footSize(2,2);

%Re-organize forces on feet
fz_lFoot   = f_lFoot(3);
taux_lFoot = f_lFoot(4);
tauy_lFoot = f_lFoot(5);
fz_rFoot   = f_rFoot(3);
taux_rFoot = f_rFoot(4);
tauy_rFoot = f_rFoot(5);

if f_lFoot(3) > Sat.toll_feetInContact && f_rFoot(3) > Sat.toll_feetInContact 
    %double support
    
    cop_lFoot  = orient_lFoot(1:2,1:2) * [-tauy_lFoot; taux_lFoot] / fz_lFoot + pose_lFoot(1:2);
    cop_rFoot  = orient_rFoot(1:2,1:2) * [-tauy_rFoot; taux_rFoot] / fz_rFoot + pose_rFoot(1:2);
    ZMP       = (fz_lFoot * cop_lFoot + fz_rFoot * cop_rFoot) / (fz_lFoot + fz_rFoot);
    
    supportPolygon_xMin = min( pose_lFoot(1), pose_rFoot(1) ) + foot_xMin;
    supportPolygon_xMax = max( pose_lFoot(1), pose_rFoot(1) ) + foot_xMax;
    supportPolygon_yMin = min( pose_lFoot(2), pose_rFoot(2) ) + foot_yMin;
    supportPolygon_yMax = max( pose_lFoot(2), pose_rFoot(2) ) + foot_yMax;
    
elseif f_lFoot(3) > Sat.toll_feetInContact
    %single support left foot
    
    cop_lFoot  = orient_lFoot(1:2,1:2) * [-tauy_lFoot; taux_lFoot] / fz_lFoot + pose_lFoot(1:2);
    ZMP       = (fz_lFoot * cop_lFoot) / (fz_lFoot);
    
    supportPolygon_xMin = pose_lFoot(1) + foot_xMin;
    supportPolygon_xMax = pose_lFoot(1) + foot_xMax;
    supportPolygon_yMin = pose_lFoot(2) + foot_yMin;
    supportPolygon_yMax = pose_lFoot(2) + foot_yMax;
    
elseif f_rFoot(3) > Sat.toll_feetInContact     
    %single support right foot
    
    cop_rFoot  = orient_rFoot(1:2,1:2) * [-tauy_rFoot; taux_rFoot] / fz_rFoot + pose_rFoot(1:2);
    ZMP       = (fz_rFoot * cop_rFoot) / (fz_rFoot);
    
    supportPolygon_xMin = pose_rFoot(1) + foot_xMin;
    supportPolygon_xMax = pose_rFoot(1) + foot_xMax;
    supportPolygon_yMin = pose_rFoot(2) + foot_yMin;
    supportPolygon_yMax = pose_rFoot(2) + foot_yMax;
    
else
    %no support
    ZMP = zeros(2,1);
    supportPolygon_xMin = 0;
    supportPolygon_xMax = 0;
    supportPolygon_yMin = 0;
    supportPolygon_yMax = 0;
end

%re-organize supportPolygon
%and add tolerance of 0.002 m on supportPolygon
supportPolygon = [supportPolygon_xMin,      supportPolygon_xMax;
                  supportPolygon_yMin-0.010, supportPolygon_yMax+0.010];

supportPolygoncenter = zeros(2,1); 
supportPolygoncenter(1) = (supportPolygon_xMax + supportPolygon_xMin)/2;
supportPolygoncenter(2) = ((supportPolygon_yMax+0.010) + (supportPolygon_yMin-0.010))/2;

zmpErr = sqrt((supportPolygoncenter(1)-ZMP(1))^2 + (supportPolygoncenter(2)-ZMP(2))^2);
